simulink model "PIDControllerTest"  (R2025b)
settings: Solver=FixedStepAuto  StartTime=0.0  StopTime=inf  FixedStep=.02  RelTol=1e-3
settings Model: Creator=ajax  LastModifiedBy=ajax

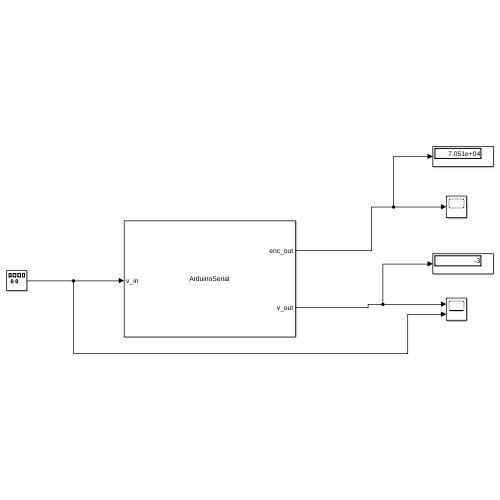
[thumbnail: Simulink's stored preview of the top-level diagram]
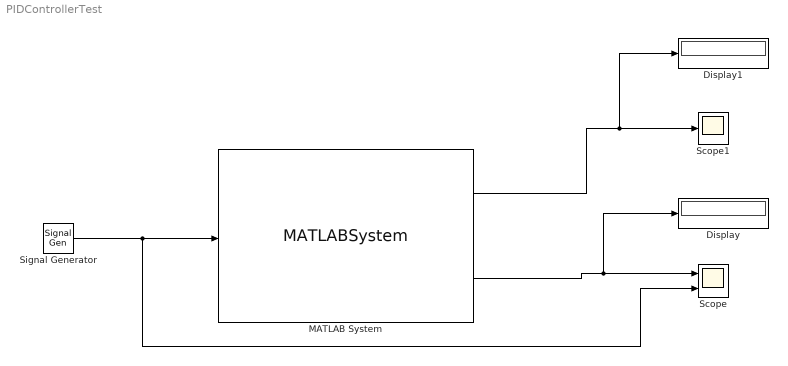
== system PIDControllerTest ==
  Display : Display
  Display1 : Display
  MATLAB System : MATLABSystem  System=ArduinoSerial  COMPort=/dev/ttyACM0  BaudRate=115200  SimulateUsing=Interpreted execution
      mask Type: ArduinoSerial
  Scope : Scope  NumInputPorts=2
      settings: ActiveDisplayYMinimum=-9.1999886149685626  ActiveDisplayYMaximum=7.3927011302915924
  Scope1 : Scope
      settings: ActiveDisplayYMinimum=-12040.874999999996  ActiveDisplayYMaximum=133827.875
  Signal Generator : SignalGenerator  WaveForm=square  Amplitude=3  Frequency=.5
  wires:
  Signal Generator/1 -> Scope/2, MATLAB System/1
  MATLAB System/2 -> Display/1, Scope/1
  MATLAB System/1 -> Display1/1, Scope1/1
